simulink model "oloop3a"  (Simulink 3.00)
settings: Solver=ode45  SolverMode=SingleTasking  StartTime=0.0  StopTime=120  MaxStep=2  RelTol=1e-3  AbsTol=1e-3
undefined symbols (not defined in the file): Aac, Bac, Cac, Dac, xinco
libraries: simulink3 x1
settings Model: SaveTime=off  SaveOutput=off  RTWTemplateMakefile=grt_vc.tmf  LastModifiedBy=Dutchroll

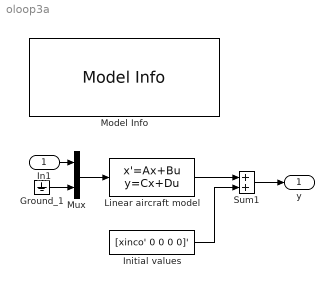
== system oloop3a ==
  In1 : Inport  Port=1  PortWidth=-1  SampleTime=-1  DataType=auto
      settings: SignalType=auto
  Ground_1 : Ground
  Initial values : Constant  Value=[xinco' 0 0 0 0]'
  Linear aircraft model : StateSpace  A=Aac  B=Bac  C=Cac  D=Dac  X0=0
  Model Info : simulink3/Signals & Systems/Model Info  InitialBlockCM=none  BlockCM=none  Frame=on  DisplayStringWithTags=|  HorizontalTextAlignment=Center  LeftAlignmentValue=0.5  SourceBlockDiagram=oloop3a  TagMaxNumber=20
      | Test system to validate linear open-
      | loop simulations of the 'Beaver'.
      | Used by OPENLOOP.M.
      | 
      | M.O. Rauw, March 2004
  Mux : Mux  Inputs=[6 6]
      settings: DisplayOption=none
  Sum1 : Sum  Inputs=++  SaturateOnIntegerOverflow=on
  y : Outport  Port=1
  wires:
  In1/1 -> Mux/1
  Ground_1/1 -> Mux/2
  Mux/1 -> Linear aircraft model/1
  Linear aircraft model/1 -> Sum1/1
  Initial values/1 -> Sum1/2
  Sum1/1 -> y/1
